simulink model "mfcPSO"  (R2015a)
settings: Solver=ode15s  StartTime=0.0  StopTime=500  RelTol=1e-9  AbsTol=1e-12
InitFcn:
  | nParticles = 2;
  | omega = 0.5;
  | 
  | dmin = 10;
  | dmax = 400;
  | 
  | T = 0.2;
  | 
  | dummy = 0;
  | 
  | dinit1 = rand * (dmax - dmin) + dmin;
  | dinit2 = rand * (dmax - dmin) + dmin;
  | 
  | %mfcInit = [5.726117682433310 0.030299840936202];
  | mfcInit1 = [2.176890899572858   0.049997860417195];
  | mfcInit2= [2.176961197280646   0.049996472695857];
settings Model: Creator=ironi  LastModifiedBy=ironi
settings HardwareCC: ProdBitPerLong=64  ProdBitPerPointer=64  ProdWordSize=64  ProdHWDeviceType=Generic->64-bit Embedded Processor (LP64)

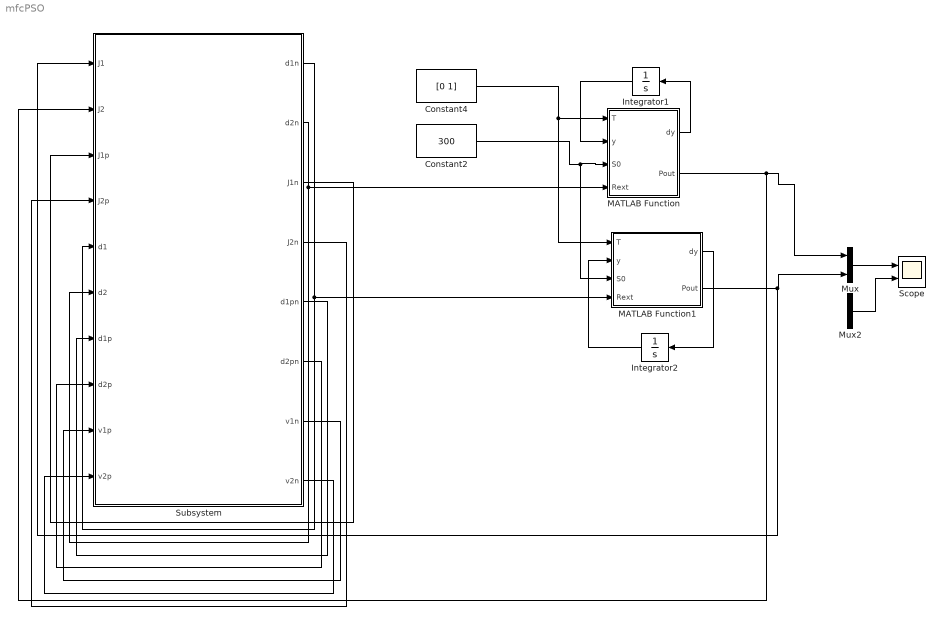
== system mfcPSO ==
  Constant2 : Constant  Value=300
  Constant4 : Constant  Value=[0 1]
  Integrator1 : Integrator  InitialCondition=mfcInit2
  Integrator2 : Integrator  InitialCondition=mfcInit1
  MATLAB Function : MATLAB Function  TreatAsAtomicUnit=on
  MATLAB Function1 : MATLAB Function  TreatAsAtomicUnit=on
  Mux : Mux  Inputs=2
  Mux2 : Mux  Inputs=2
  Scope : Scope  NumInputPorts=2
      settings: YMin=0.00172~147  YMax=0.001734~168
  Subsystem : Subsystem
  wires:
  Mux/1 -> Scope/1
  MATLAB Function/1(dy) -> Integrator1/1
  Mux2/1 -> Scope/2
  MATLAB Function1/2(Pout) -> Subsystem/1(J1), Mux/2
  MATLAB Function/2(Pout) -> Subsystem/2(J2), Mux/1
  Integrator1/1 -> MATLAB Function/2(y)
  MATLAB Function1/1(dy) -> Integrator2/1
  Constant4/1 -> MATLAB Function/1(T), MATLAB Function1/1(T)
  Constant2/1 -> MATLAB Function/3(S0), MATLAB Function1/3(S0)
  Integrator2/1 -> MATLAB Function1/2(y)
  Subsystem/1(d1n) -> MATLAB Function1/4(Rext), Subsystem/5(d1)
  Subsystem/2(d2n) -> MATLAB Function/4(Rext), Subsystem/6(d2)
  Subsystem/5(d1pn) -> Subsystem/7(d1p)
  Subsystem/6(d2pn) -> Subsystem/8(d2p)
  Subsystem/7(v1n) -> Subsystem/9(v1p)
  Subsystem/8(v2n) -> Subsystem/10(v2p)
  Subsystem/3(J1n) -> Subsystem/3(J1p)
  Subsystem/4(J2n) -> Subsystem/4(J2p)

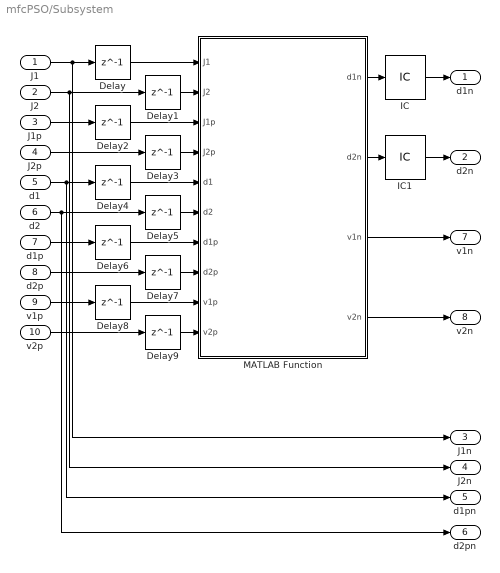
== system mfcPSO/Subsystem ==
  J1 : Inport
  J2 : Inport  Port=2
  J1p : Inport  Port=3
  J2p : Inport  Port=4
  d1 : Inport  Port=5
  d2 : Inport  Port=6
  d1p : Inport  Port=7
  d2p : Inport  Port=8
  v1p : Inport  Port=9
  v2p : Inport  Port=10
  Delay{,1..9} (10 alike) : Delay  DelayLength=1  InitialCondition=0  SampleTime=T
  IC : InitialCondition  Value=dinit1
  IC1 : InitialCondition  Value=dinit2
  MATLAB Function : MATLAB Function  TreatAsAtomicUnit=on
  d1n : Outport
  d2n : Outport  Port=2
  J1n : Outport  Port=3
  J2n : Outport  Port=4
  d1pn : Outport  Port=5
  d2pn : Outport  Port=6
  v1n : Outport  Port=7
  v2n : Outport  Port=8
  wires:
  J1/1 -> J1n/1, Delay/1
  MATLAB Function/2(d2n) -> IC1/1
  MATLAB Function/1(d1n) -> IC/1
  Delay/1 -> MATLAB Function/1(J1)
  Delay1/1 -> MATLAB Function/2(J2)
  Delay2/1 -> MATLAB Function/3(J1p)
  Delay3/1 -> MATLAB Function/4(J2p)
  Delay4/1 -> MATLAB Function/5(d1)
  Delay5/1 -> MATLAB Function/6(d2)
  Delay6/1 -> MATLAB Function/7(d1p)
  Delay7/1 -> MATLAB Function/8(d2p)
  Delay8/1 -> MATLAB Function/9(v1p)
  Delay9/1 -> MATLAB Function/10(v2p)
  IC/1 -> d1n/1
  IC1/1 -> d2n/1
  J2/1 -> J2n/1, Delay1/1
  J1p/1 -> Delay2/1
  J2p/1 -> Delay3/1
  d1/1 -> d1pn/1, Delay4/1
  d2/1 -> d2pn/1, Delay5/1
  d1p/1 -> Delay6/1
  d2p/1 -> Delay7/1
  v1p/1 -> Delay8/1
  v2p/1 -> Delay9/1
  MATLAB Function/3(v1n) -> v1n/1
  MATLAB Function/4(v2n) -> v2n/1

== matlab function mfcPSO/MATLAB Function1 ==
  data: T input; dy output; y input; dummy parameter; S0 input; Rext input; Pout output
function [dy, Pout]= mfcModelFast(T, y, dummy, S0, Rext)
F = 96485;%
R = 8.314472;%
T = 298.15;%
yield = 22.753;%
% Ych4 = .3;%
qmax_a = 8.484;%
qmax_m = 8.2;%
umax_a = 1.9753;%
umax_m = .1;%
Ks_a = 20;%
Ks_m = 80;%
m = 2;%
gamma = 663400;%
Mtotal = .05;%
Km = .2*Mtotal;%
% Kd_a = .02*umax_a;%
% Kd_m = .02*umax_m;%
Xmax = 512.5;%
Kx = .01*4;%
Rmin = 25;%
Rmax = 2000 + Rmin;%
Emin = .01;%
Emax = 0.25 + 0.4144+ Emin;%
Kr = .024;%

% i0ref=0.4*4;%

e = 0.0001*Mtotal;%

V = 0.2;%
Fin = 0.1527;%

D = Fin/V;

Xtot = 500;

Xeg = 250;

S   = y(1);
Mox = y(2);
xm = Xtot - Xeg;


%% Équations dynamiques
  
Mred = Mtotal - Mox;

Rint = Rmin + (Rmax - Rmin) * exp(-Kr*Xeg);                         % (22)
Eocv = Emin + (Emax - Emin) * exp(-1/(Kr*Xeg));                     % (23)

% alpha = 1/2*(1 + tanh(Kx*(Xeg + xm - Xmax)));                    % (9)

qa = qmax_a * S / (Ks_a + S) * Mox / (Km + Mox);                    % (15)
qm = qmax_m * S / (Ks_m + S);                                       % (16)

% ueg = umax_a * S / (Ks_a + S) * Mox / (Km + Mox);                    % (13)

% Imfc = (Eocv - n_conc) / (Rext + Rint) * Mred / (e + Mred);         % (21)
temp = Eocv - (R*T/m/F)*abs(log(complex(Mtotal/Mred)));
% Imfc = (Eocv - (R*T/m/F)*abs(log(complex(Mtotal/Mred))))/(Rext+Rint)*Mred/(e+Mred);
Imfc = temp/(Rext+Rint)*Mred/(e+Mred);

% Pout = ((Eocv - (R*T/m/F)*abs(log(complex(Mtotal/Mred))))*Mred/(e+Mred)-Rint*Imfc)*Imfc;
Pout = (temp*Mred/(e+Mred)-Rint*Imfc)*Imfc;

Sp = -qa*Xeg - qm*xm + D*(S0 - S);                                   % (6)
% Xap = ueg*xa - Kd_a*xa - alpha_a*D*xa;                               % (7)
% Xmp = um*xm - Kd_m*xm - alpha_m*D*xm;                               % (8)

Moxp = -yield*qa + gamma*Imfc / (m*F*V*Xeg) * 86400;                 % (12)

% if xa < 1 && Xap < 0
%   Xap = 0;
% end
% 
% if xm < 0.99 && Xmp < 0
%   Xmp = 0;
% end

% Pout = Rext*Imfc^2;

% dy = [Sp; Xap; Xmp; Moxp];
dy = [Sp; Moxp];

== matlab function mfcPSO/MATLAB Function ==
  data: T input; dy output; y input; dummy parameter; S0 input; Rext input; Pout output
function [dy, Pout]= mfcModelFast(T, y, dummy, S0, Rext)
F = 96485;%
R = 8.314472;%
T = 298.15;%
yield = 22.753;%
% Ych4 = .3;%
qmax_a = 8.484;%
qmax_m = 8.2;%
umax_a = 1.9753;%
umax_m = .1;%
Ks_a = 20;%
Ks_m = 80;%
m = 2;%
gamma = 663400;%
Mtotal = .05;%
Km = .2*Mtotal;%
% Kd_a = .02*umax_a;%
% Kd_m = .02*umax_m;%
Xmax = 512.5;%
Kx = .01*4;%
Rmin = 25;%
Rmax = 2000 + Rmin;%
Emin = .01;%
Emax = 0.25 + 0.4144+ Emin;%
Kr = .024;%

% i0ref=0.4*4;%

e = 0.0001*Mtotal;%

V = 0.2;%
Fin = 0.1527;%

D = Fin/V;

Xtot = 500;

Xeg = 250;

S   = y(1);
Mox = y(2);
xm = Xtot - Xeg;


%% Équations dynamiques
  
Mred = Mtotal - Mox;

Rint = Rmin + (Rmax - Rmin) * exp(-Kr*Xeg);                         % (22)
Eocv = Emin + (Emax - Emin) * exp(-1/(Kr*Xeg));                     % (23)

% alpha = 1/2*(1 + tanh(Kx*(Xeg + xm - Xmax)));                    % (9)

qa = qmax_a * S / (Ks_a + S) * Mox / (Km + Mox);                    % (15)
qm = qmax_m * S / (Ks_m + S);                                       % (16)

% ueg = umax_a * S / (Ks_a + S) * Mox / (Km + Mox);                    % (13)

% Imfc = (Eocv - n_conc) / (Rext + Rint) * Mred / (e + Mred);         % (21)
temp = Eocv - (R*T/m/F)*abs(log(complex(Mtotal/Mred)));
% Imfc = (Eocv - (R*T/m/F)*abs(log(complex(Mtotal/Mred))))/(Rext+Rint)*Mred/(e+Mred);
Imfc = temp/(Rext+Rint)*Mred/(e+Mred);

% Pout = ((Eocv - (R*T/m/F)*abs(log(complex(Mtotal/Mred))))*Mred/(e+Mred)-Rint*Imfc)*Imfc;
Pout = (temp*Mred/(e+Mred)-Rint*Imfc)*Imfc;

Sp = -qa*Xeg - qm*xm + D*(S0 - S);                                   % (6)
% Xap = ueg*xa - Kd_a*xa - alpha_a*D*xa;                               % (7)
% Xmp = um*xm - Kd_m*xm - alpha_m*D*xm;                               % (8)

Moxp = -yield*qa + gamma*Imfc / (m*F*V*Xeg) * 86400;                 % (12)

% if xa < 1 && Xap < 0
%   Xap = 0;
% end
% 
% if xm < 0.99 && Xmp < 0
%   Xmp = 0;
% end

% Pout = Rext*Imfc^2;

% dy = [Sp; Xap; Xmp; Moxp];
dy = [Sp; Moxp];

== matlab function mfcPSO/Subsystem/MATLAB Function ==
  data: J1 input; d1n output; J2 input; J1p input; J2p input; d1 input; d2 input; d1p input; d2p input; v1p input; v2p input; d2n output; v1n output; v2n output
function [d1n,d2n, v1n, v2n]= fcn(J1,J2,J1p,J2p,d1,d2,d1p,d2p,v1p,v2p)
%#codegen

dmin = 10;
dmax = 400;
omega = 0.5;

c1 = 2;
c2 = 3;

MaxOfUnits = max(J1,J2);

MaxVal1 = max(J1,J1p);
MaxVal2 = max(J2,J2p);

if MaxVal1 == J1
  Pbest1 = d1;
else
  Pbest1 = d1p;
end

if MaxVal2 == J2
  Pbest2 = d2;
else
  Pbest2 = d2p;
end

if MaxOfUnits == J1
  Gbest = d1;
else
  Gbest = d2;
end

v1 = (omega * v1p) + (c1*rand*(Pbest1-d1)) + (c2*rand*(Gbest-d1));
v2 = (omega * v2p) + (c1*rand*(Pbest2-d2)) + (c2*rand*(Gbest-d2));

d1n = d1 + v1;
if d1n > dmax
  d1n = dmax;
elseif d1n < dmin
  d1n = dmin;
end

d2n = d2 + v2;
if d2n > dmax
  d2n = dmax;
elseif d2n < dmin
  d2n = dmin;
end
